simulink model "Simulation"  (R2019a)
settings: Solver=VariableStepAuto  StartTime=0.0  StopTime=10.0  RelTol=1e-3
settings Model: Creator=liamh  LastModifiedBy=liamh

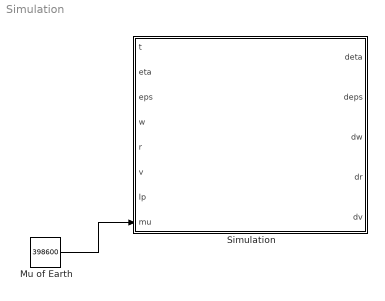
== system Simulation ==
  "Mu of Earth " : Constant  Value=398600
  Simulation : MATLAB Function  TreatAsAtomicUnit=on
  wires:
  "Mu of Earth "/1 -> Simulation/8(mu)

== matlab function Simulation/Simulation ==
  data: t input; deta output; eta input; eps input; w input; r input; v input; Ip input; mu input; deps output; dw output; dr output; dv output
function [ deta , deps , dw , dr , dv ]   = Simulation( t , eta , eps , w , r , v , Ip , mu )
% ( t , eta , eps , w , r , v , Ip , Avec , Day0 , mbar , UTC , mu)
% Simulates an attitude of s/c in LEO. State is quaternion [ eta , eps ]
% followed by angular velocity

% to track progress
t ;

% Set up names
    Ix = Ip(1,1) ;
    Iy = Ip(2,2) ;
    Iz = Ip(3,2) ;
%     Ax = Avec(1) ;
%     Ay = Avec(2) ;
%     Az = Avec(3) ;

%     Cbg = quat2dcm( [ eta , eps' ] ) ;
    
%      % FIX THIS
%      if t >= 60
%          tmin = floor( t/60 ) ;
%          t = t - tmin*60 ;
%          if tmin >= 60
%              thour = floor( tmin/60 ) ;
%              tmin = tmin - thour*60 ;
%          else
%              thour = 0 ;
%          end
%      else
%          tmin = 0 ;
%          thour = 0 ;
%      end
%      UTCnow = UTC + [ 0 0 0 thour tmin t ] ;

%     JDay = Day0 + t/(24*60*60) ; % Find Julian day of current moment
%     JYear = JDay/365.2422 ; % Find Julian year 
%     [ rerels , ~ ] = planetary_state(3,JYear) ; %Find position vector of earth relative to the sun

% Find change in quaternions
        epscross = crossmatrix( eps ) ;
    epsdot = .5 * ( eta*eye(3) + epscross ) * w ;
    etadot = .5 * eps * w ;
    
% % Find sun unit vector
%     theta = 23.4 ; % angle between ecliptic and equitorial plane
%     Cs2eci = [ 1 0 0 ; 0 cosd(theta) sind(theta) ; 0 -sin(theta) cos(theta) ] ; % rotation about x-axis
%     rsun = - Cs2eci*rerels ; % find sun direction in eci by taking the negative of the earth position vector rotated to equitorial plane about first point of aries
%     s = rsun/norm(rsun) ; % make sun vector a unit vector
%     directs = dot( s , r/norm(r) ) ; % similarity in direction of satellite and sun direction
%     if directs >= -.3 
%         s = s ;
%     else
%         s = 0 ;
%     end
    
% % Find torques
%      Tsrp = SolarRadiationPressure( Cbg , s , Ax , Ay , Az ) ;
%      Tgg = GravityGradientTorque( Cbg , Ix , Iy , Iz , r ) ;
% %    Tmag = MagneticTorque( Cbg , mbar , r , UTCnow ) ;
%     
%     T = Tsrp+Tgg;
% %     T = Tsrp + Tgg + Tmag ;
    
% Find change in angular velocity from torques 
    wdot = zeros( 3,1 ) ;
    wdot(1) = (T(1)-( Iz - Iy )*w(2)*w(3))/Ix ;
    wdot(2) = (T(2)-( Ix - Iz )*w(1)*w(3))/Iy ;
    wdot(3) = (T(3)-( Iy - Ix )*w(2)*w(1))/Iz ;
    
% New ECI state vectors
    rad = norm( r ) ; %radius
    rdot = v ;
    vdot = -mu*r/rad^3 ;

%     function [ r , v ] = planetary_state(planet_id,T)
%     % Planetary Ephemerides from Meeus (1991:202-204) and J2000.0
%     % Output:
%     % planet_coes
%     % a = semimajor axis (km)
%     % ecc = eccentricity
%     % inc = inclination (degrees)
%     % raan = right ascension of the ascending node (degrees)
%     % w_hat = longitude of perihelion (degrees)
%     % L = mean longitude (degrees)
% 
%     % Inputs:
%     % planet_id - planet identifier:
%     % 1 = Mercury
%     % 2 = Venus
%     % 3 = Earth
%     % 4 = Mars
%     % 5 = Jupiter
%     % 6 = Saturn
%     % 7 = Uranus
%     % 8 = Neptune
% 
%     if planet_id == 1
%         a = 0.387098310; % AU but in km later
%         ecc = 0.20563175 + 0.000020406*T - 0.0000000284*T^2 - 0.00000000017*T^3;
%         inc = 7.004986 - 0.0059516*T + 0.00000081*T^2 + 0.000000041*T^3; %degs
%         raan = 48.330893 - 0.1254229*T-0.00008833*T^2 - 0.000000196*T^3; %degs
%         w_hat = 77.456119 +0.1588643*T -0.00001343*T^2+0.000000039*T^3; %degs
%         L = 252.250906+149472.6746358*T-0.00000535*T^2+0.000000002*T^3; %degs
%     elseif planet_id == 2
%         a = 0.723329820; % AU
%         ecc = 0.00677188 - 0.000047766*T + 0.000000097*T^2 + 0.00000000044*T^3;
%         inc = 3.394662 - 0.0008568*T - 0.00003244*T^2 + 0.000000010*T^3; %degs
%         raan = 76.679920 - 0.2780080*T-0.00014256*T^2 - 0.000000198*T^3; %degs
%         w_hat = 131.563707 +0.0048646*T -0.00138232*T^2-0.000005332*T^3; %degs
%         L = 181.979801+58517.8156760*T+0.00000165*T^2-0.000000002*T^3; %degs
%     elseif planet_id == 3 
%         a = 1.000001018; % AU
%         ecc = 0.01670862 - 0.000042037*T - 0.0000001236*T^2 + 0.00000000004*T^3;
%         inc = 0.0000000 + 0.0130546*T - 0.00000931*T^2 - 0.000000034*T^3; %degs
%         raan = 0.0; %degs
%         w_hat = 102.937348 + 0.3225557*T + 0.00015026*T^2 + 0.000000478*T^3; %degs
%         L = 100.466449 + 35999.372851*T - 0.00000568*T^2 + 0.000000000*T^3; %degs
%     elseif planet_id == 4
%         a = 1.523679342; % AU
%         ecc = 0.09340062 + 0.000090483*T - 0.00000000806*T^2 - 0.00000000035*T^3;
%         inc = 1.849726 - 0.0081479*T - 0.00002255*T^2 - 0.000000027*T^3; %degs
%         raan = 49.558093 - 0.2949846*T-0.00063993*T^2 - 0.000002143*T^3; %degs
%         w_hat = 336.060234 +0.4438898*T -0.00017321*T^2+0.000000300*T^3; %degs
%         L = 355.433275+19140.2993313*T+0.00000261*T^2-0.000000003*T^3; %degs
%     elseif planet_id == 5
%         a = 5.202603191 + 0.0000001913*T; % AU
%         ecc = 0.04849485+0.000163244*T - 0.0000004719*T^2 + 0.00000000197*T^3;
%         inc = 1.303270 - 0.0019872*T + 0.00003318*T^2 + 0.000000092*T^3; %degs
%         raan = 100.464441 + 0.1766828*T+0.00090387*T^2 - 0.000007032*T^3; %degs
%         w_hat = 14.331309 +0.2155525*T +0.00072252*T^2-0.000004590*T^3; %degs
%         L = 34.351484+3034.9056746*T-0.00008501*T^2+0.000000004*T^3; %degs
%     elseif planet_id == 6
%         a = 9.5549009596 - 0.0000021389*T; % AU
%         ecc = 0.05550862 - 0.000346818*T -0.0000006456*T^2 + 0.00000000338*T^3;
%         inc = 2.488878 + 0.0025515*T - 0.00004903*T^2 + 0.000000018*T^3; %degs
%         raan = 113.665524 - 0.2566649*T-0.00018345*T^2 + 0.000000357*T^3; %degs
%         w_hat = 93.056787 +0.5665496*T +0.00052809*T^2-0.000004882*T^3; %degs
%         L = 50.077471+1222.1137943*T+0.00021004*T^2-0.000000019*T^3; %degs
%     elseif planet_id == 7
%         a = 19.218446062-0.0000000372*T+0.00000000098*T^2; % AU
%         ecc = 0.04629590 - 0.000027337*T + 0.0000000790*T^2 + 0.00000000025*T^3;
%         inc = 0.773196 - 0.0016869*T + 0.00000349*T^2 + 0.00000000016*T^3; %degs
%         raan = 74.005947 + 0.0741461*T+0.00040540*T^2 +0.000000104*T^3; %degs
%         w_hat = 173.005159 +0.0893206*T -0.00009470*T^2+0.000000413*T^3; %degs
%         L = 314.055005+428.4669983*T-0.00000486*T^2-0.000000006*T^3; %degs
%     elseif planet_id == 8
%         a = 30.110386869-0.0000001663*T+0.00000000069*T^2; % AU
%         ecc = 0.00898809 + 0.000006408*T -0.0000000008*T^2;
%         inc = 1.769952 +0.0002557*T +0.00000023*T^2 -0.0000000000*T^3; %degs
%         raan = 131.784057 - 0.0061651*T-0.00000219*T^2 - 0.000000078*T^3; %degs
%         w_hat = 48.123691 +0.0291587*T +0.00007051*T^2-0.000000000*T^3; %degs
%         L = 304.348665+218.4862002*T+0.00000059*T^2-0.000000002*T^3; %degs
%     end
% 
%     planet_coes = [a;ecc;inc;raan;w_hat;L];
%     %Convert to km:
%     au = 149597870;
%     planet_coes(1) = planet_coes(1)*au;
%     mus = 1.32712440018e20 ;
%     [ r , v ] = Pcoes2state( planet_coes , mus ) ;
% 
%         function [ r , v ] = Pcoes2state( p_coes , mu )
%                 d2r = pi/180 ;
%                 h = sqrt( p_coes(1)*mu*(1-p_coes(2)^2) ) ;
%                 omega = p_coes(6) - p_coes(4) ;
%                 M = p_coes(6)*d2r - p_coes(5)*d2r ;
%                 T = (2*pi)/sqrt(mu)*p_coes(1) ;
%                 t = M*T/(2*pi) ;
%                 [ theta ] = time2theta( t , T , p_coes(2) ) ;
%                 [ r , v ] = coes2state(  h , p_coes(2) , theta , p_coes(4) , omega , p_coes(3) , mu ) ;
% 
%             function [ theta ] = time2theta( t , T , ecc )
%             % Find true anomaly at a time
% 
%             n = 2*pi/T ; % mean motion
%             Me = n*t ; 
% 
%             % Guess of E
%             if Me < pi
%                 E0 = Me + ecc/2 ;
%             else
%                 E0 = Me - ecc/2 ;
%             end
% 
%             % Use Newtons to find E
%                 tol = 10^-8 ; % Tolerance
%                 lim = 1000 ; % Maximum iteration
%                 f = @(E) E - ecc*sin(E) - Me ; % Function handle for E
%                 fprime = @(E) 1 - ecc*cos(E) ; % function handle for derivative of E
%                 [ E ] = newton( E0 , f , fprime , tol , lim ) ; % Apply Newtons
% 
%             theta = 2*atan(tan(E/2)*sqrt((1+ecc)/(1-ecc))) ; % find true anomaly
%             % correction to make it positive
%                 if theta < 0
%                     theta = theta + 2*pi ;
%                 end
%             theta = theta*(180/pi) ;
%             end
%             function [ r , v ] = coes2state(  h , ecc , theta , RAAN , omega , inc , mu )
%                 r_peri = (h^2/mu) * ( 1/( 1 + ecc*cosd(theta) ) ) * [ cosd( theta ) ; sind( theta ) ; 0 ] ;
%                 v_peri = (mu/h) * [ -sind( theta ) ; ecc+cosd(theta) ; 0 ] ;
% 
%                 d2r = pi/180 ;
%                 RAAN = d2r*RAAN ;
%                 omega = d2r*omega ;
%                 inc = d2r*inc ;
%                 Q(1,1) = -sin(RAAN)*cos(inc)*sin(omega) + cos(RAAN)*cos(omega) ;
%                 Q(1,2) = -sin(RAAN)*cos(inc)*cos(omega) - cos(RAAN)*sin(omega) ;
%                 Q(1,3) = sin(RAAN)*sin(inc) ;
%                 Q(2,1) = cos(RAAN)*cos(inc)*sin(omega) + sin(RAAN)*cos(omega) ;
%                 Q(2,2) = cos(RAAN)*cos(inc)*cos(omega) - sin(RAAN)*sin(omega) ;
%                 Q(2,3) = -cos(RAAN)*sin(inc) ;
%                 Q(3,1) = sin(inc)*sin(omega) ;
%                 Q(3,2) = sin(inc)*cos(omega) ;
%                 Q(3,3) = cos(inc) ;
% 
%                 r = Q*r_peri ;
%                 v = Q*v_peri ;
%             end
%         end
%         function [ x ] = newton( x0 , f , fprime , tol , lim )
%         % Uses Newtons Method to find x given initial guess x0, function f,
%         % derivative fprime, tolerance tol, and limit on the iterations lim
% 
%             x = x0 ;
%             ii = 1 ;
%             ratio = 1 ;
%                 while abs(ratio(ii)) >= tol
%                     ratio(ii+1) = f(x(ii))/fprime(x(ii)) ;
%                     x(ii+1) = x(ii) - ratio(ii+1) ;
%                     ii = ii + 1 ;
%                         if ii > lim
%                             error([ 'Ran ' , num2str( lim ) , ' times without a solution' ])
%                         end
%                 end
%         x = x( ii ) ;
%         end
%     end % Planetary COES is from Dr. A, State conversion code is mine
% 
% end
